simulink model "reconstruction_block"  (R2021a)
settings: Solver=VariableStepAuto  StartTime=0.0  StopTime=10.0  RelTol=1e-3
settings Model: Creator=yadu1  LastModifiedBy=sumuk

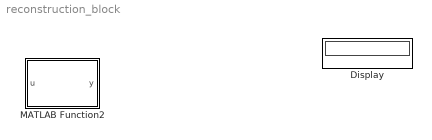
== system reconstruction_block ==
  Display : Display
  MATLAB Function2 : MATLAB Function  TreatAsAtomicUnit=on

== matlab function reconstruction_block/MATLAB Function2 ==
  data: u input; y output
function y = idct(u)

y = u;
